simulink model "Lab_6_Task_2"  (R2022b)
settings: Solver=VariableStepAuto  StartTime=0.0  StopTime=10.0  RelTol=1e-3
settings Model: Creator=Azlaan  LastModifiedBy=Azlaan

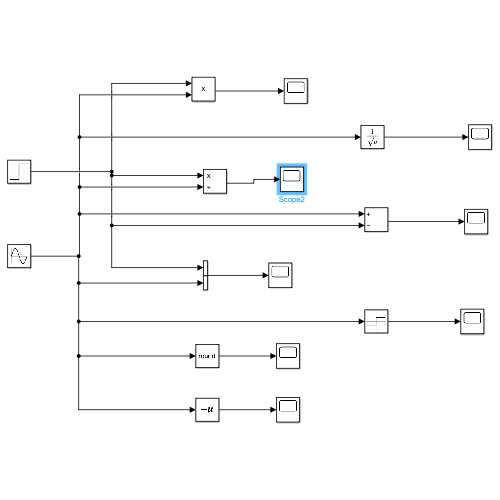
[thumbnail: Simulink's stored preview of the top-level diagram]
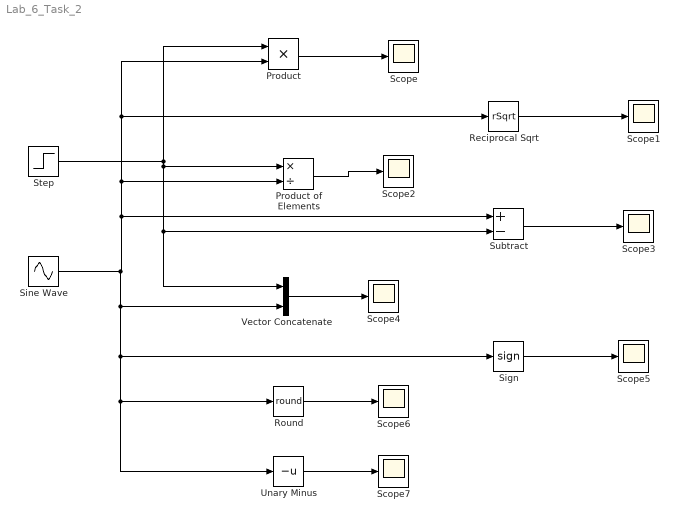
== system Lab_6_Task_2 ==
  Product : Product
  Product of Elements : Product  Inputs=*/
  Reciprocal Sqrt : Sqrt  Operator=rSqrt
  Round : Rounding  Operator=round
  Scope{,1..7} (8 alike) : Scope
  Sign : Signum
  Sine Wave : Sin  SampleTime=0
  Step : Step  SampleTime=0
  Subtract : Sum  Inputs=+-
  Unary Minus : UnaryMinus
  Vector Concatenate : Concatenate
  wires:
  Product/1 -> Scope/1
  Step/1 -> Product of Elements/1, Vector Concatenate/1, Subtract/2, Product/1
  Reciprocal Sqrt/1 -> Scope1/1
  Product of Elements/1 -> Scope2/1
  Sine Wave/1 -> Unary Minus/1, Round/1, Sign/1, Vector Concatenate/2, Product/2, Reciprocal Sqrt/1, Product of Elements/2, Subtract/1
  Subtract/1 -> Scope3/1
  Vector Concatenate/1 -> Scope4/1
  Sign/1 -> Scope5/1
  Round/1 -> Scope6/1
  Unary Minus/1 -> Scope7/1
